simulink model "Constant_vel"  (R2024b)
settings: Solver=FixedStepAuto  StartTime=0.0  StopTime=10  FixedStep=0.001  RelTol=1e-3
libraries: simulink x2
settings Model: Creator=cpero  LastModifiedBy=cpero

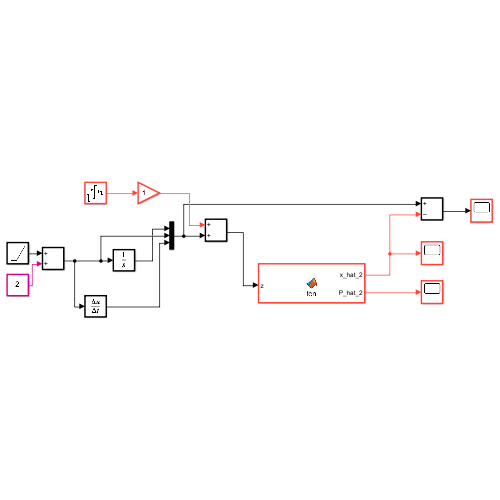
[thumbnail: Simulink's stored preview of the top-level diagram]
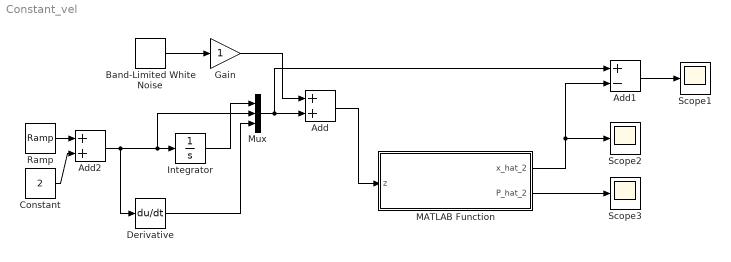
== system Constant_vel ==
  Add : Sum
  Add1 : Sum  Inputs=+-
  Add2 : Sum
  Band-Limited White Noise : simulink/Sources/Band-Limited White Noise  Cov=[1e-3 1e-3 1e-3]  Ts=0.001  seed=[1 2 3]
  Constant : Constant  Value=2
  Derivative : Derivative
  Gain : Gain
  Integrator : Integrator  InitialCondition=-1
  MATLAB Function : MATLAB Function  TreatAsAtomicUnit=on
  Mux : Mux  Inputs=3
  Ramp : simulink/Sources/Ramp  slope=1  start=0  InitialOutput=1
  Scope1 : Scope
  Scope2 : Scope
  Scope3 : Scope
  wires:
  Add2/1 -> Derivative/1, Mux/2, Integrator/1
  Integrator/1 -> Mux/1
  Mux/1 -> Add1/1, Add/2
  Band-Limited White Noise/1 -> Gain/1
  Gain/1 -> Add/1
  MATLAB Function/1(x_hat_2) -> Add1/2, Scope2/1
  MATLAB Function/2(P_hat_2) -> Scope3/1
  Add1/1 -> Scope1/1
  Add/1 -> MATLAB Function/1(z)
  Ramp/1 -> Add2/1
  Constant/1 -> Add2/2
  Derivative/1 -> Mux/3

== matlab function Constant_vel/MATLAB Function ==
  settings: updateMethod=DISCRETE
  data: z input; x_hat_2 output; P_hat_2 output
function [x_hat_2, P_hat_2] = fcn(z)

persistent x_hat_2_prior P_hat_2_prior

time_step = 1e-3;

F = [1 time_step 0.5*time_step^2;
     0 1 time_step
     0 0 1];
H = eye(3);
Q = zeros(3);
R = eye(3);

if isempty(x_hat_2_prior)
    x_hat_2_prior = [0;0;0];
    P_hat_2_prior = [1 0 0;
                     0 1 0;
                     0 0 1];
end

%Predict
x_hat_1 = F*x_hat_2_prior;
P_hat_1 = F*P_hat_2_prior*F' + Q;

%Update
y = z - H*x_hat_1;
S = H*P_hat_1*H' + R;
K = P_hat_1*H'*inv(S);
x_hat_2 = x_hat_1 + K*y;
P_hat_2 = (eye(3) - K*H)*P_hat_1;

x_hat_2_prior = x_hat_2;
P_hat_2_prior = P_hat_2;
